simulink model "testPVAsset"  (R2012b)
settings: Solver=FixedStepDiscrete  StartTime=0.0  StopTime=86400  FixedStep=10  RelTol=1e-3
libraries: simulink x1, DiSC_ToolboxOpal_V11 x1
settings Model: Creator=rlo  LastModifiedBy=smartgrid
settings DataIOCC: SignalLoggingSaveFormat=ModelDataLogs
settings OptimizationCC: ExpressionDepthLimit=128
settings DebuggingCC: UnderspecifiedInitializationDetection=Simplified  MergeDetectMultiDrivingBlocksExec=error  MultiTaskDSMMsg=warning  MultiTaskCondExecSysMsg=none  StateNameClashWarn=none  StrictBusMsg=ErrorOnBusTreatedAsVector
settings RTWCC: IncludeERTFirstTime=on
settings CodeAppCC: CustomSymbolStrType=$N$R$M_T  InternalIdentifier=Shortened
settings GRTTargetCC: CodeReplacementLibrary=None  CPPClassGenCompliant=on

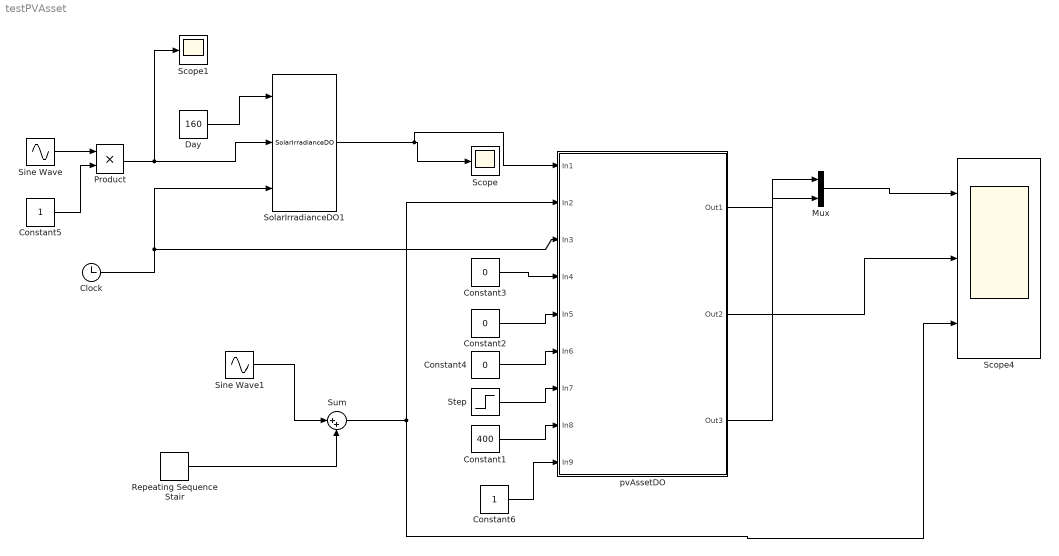
== system testPVAsset ==
  Clock : Clock
  Constant1 : Constant  Value=400
  Constant2 : Constant  Value=0
  Constant3 : Constant  Value=0
  Constant4 : Constant  Value=0
  Constant5 : Constant
  Constant6 : Constant
  Day : Constant  Value=160
  Mux : Mux  Inputs=2
  Product : Product
  Repeating Sequence Stair : simulink/Sources/Repeating Sequence Stair  OutValues="10*[3*ones(1,100)  1*ones(1,100) 4*ones(1,100) 2*ones(1,100) 1*ones(1,100)].'"  tsamp=-1  OutMin=[]  OutMax=[]  OutDataTypeStr=double  OutputDataTypeScalingMode=double  OutDataType=fixdt(0,8)  ConRadixGroup=Best Precision: Vector-wise  OutScaling=2^-12
  Scope : Scope
      settings: YMin=0  YMax=1600
  Scope1 : Scope
      settings: YMin=0  YMax=1
  Scope4 : Scope  NumInputPorts=3
      settings: YMin=0~-5~-5  YMax=6000~5~5  SaveName=ScopeData4
  Sine Wave : Sin  Amplitude=0.5  Bias=0.5  Frequency=0.00004  Phase=pi
  Sine Wave1 : Sin  Amplitude=30  Bias=400  Frequency=0.0001  Phase=pi  SampleTime=0
  SolarIrradianceDO1 : DiSC_ToolboxOpal_V11/SolarIrradianceDO
  Step : Step  Time=0  After=2  SampleTime=0
  Sum : Sum  Inputs=|++
  pvAssetDO : Subsystem
      mask help:
      | %pvAssetDO implements a simple P,Q controllable solar PV system using MATLAB embedded function.
      |     %   The pvAsset can be set to follow an active power reference, output
      |     %   maximum power available or derate power. It can also, at the same
      |     %   time be set to follow a reactive power reference, output the
      |     %   minimum reactive power according to the power factor or try to keep
      |     %   a voltage reference in the coupling point by controlling reactive
      |     %   power output.
      |     %
      |     %
      |     % Revision:
      |     % 19-06-2014, R. Pedersen, Aalborg University. Notes:
      |     % R. Pedersen 11-6-2014, Aalborg University
      |     % 29-11-2014, R. Olsen/M. Kemal, Aalborg University (Simulink)
      |     % 20-06-2015, F. Iov/M. Kemal, Aalborg University (Simulink toolbox for OPAL)
      |
      |                 % Input:
      |             %   - s [w/m^2], is the solar irradiance.
      |             %   - v [V], is the voltage at the connection point.
      |             %   - dP [PU], is the reference to active power change (curtailment).
      |             %   - dPlim [PU], is the reference to derated power (derate)
      |             %   - qRef [VAR], is the reactive power reference.
      |             %   - vRef [V], is the voltage reference.
      |             %
      |             % Output:
      |             %   - p [W], is the active power output
      |             %   - q [VAR], is the reactive power output
      |             %   - pAva [W], is the available power
      mask Help:
      | %pvAssetDO implements a simple P,Q controllable solar PV system using MATLAB embedded function.
      |     %   The pvAsset can be set to follow an active power reference, output
      |     %   maximum power available or derate power. It can also, at the same
      |     %   time be set to follow a reactive power reference, output the
      |     %   minimum reactive power according to the power factor or try to keep
      |     %   a voltage reference in the coupling point by controlling reactive
      |     %   power output.
      |     %
      |     %
      |     % Revision:
      |     % 19-06-2014, R. Pedersen, Aalborg University. Notes:
      |     % R. Pedersen 11-6-2014, Aalborg University
      |     % 29-11-2014, R. Olsen/M. Kemal, Aalborg University (Simulink)
      |     % 20-06-2015, F. Iov/M. Kemal, Aalborg University (Simulink toolbox for OPAL)
      | 
      |                 % Input:
      |             %   - s [w/m^2], is the solar irradiance.
      |             %   - v [V], is the voltage at the connection point.
      |             %   - dP [W], is the reference to active power change.
      |             %   - dPlim [W], is the reference to derated power.
      |             %   - qRef [VAR], is the reactive power reference.
      |             %   - vRef [V], is the voltage reference.
      |             %
      |             % Output:
      |             %   - p [W], is the active power output
      |             %   - q [VAR], is the reactive power output
      |             %   - pAva [W], is the available power
      mask Display:
      | image(imread( 'PhotoVoltaic.png'))
      | port_label( 'output',1, 'p')
      | port_label( 'output',2, 'q')
      | port_label( 'output',3, 'pAva')
      | 
      | 
      | port_label( 'input',1, 'solarIrr')
      | port_label( 'input',2, 'vMeas')
      | port_label( 'input',3, 'time')
      | port_label( 'input',4, 'dp')
      | port_label( 'input',5, 'dplim')
      | port_label( 'input',6, 'qRef')
      | port_label( 'input',7, 'qMode')
      | port_label( 'input',8, 'vRef')
      | port_label( 'input',9, 'pMode')
  wires:
  SolarIrradianceDO1/1 -> pvAssetDO/1(In1), Scope/1
  Day/1 -> SolarIrradianceDO1/1
  Clock/1 -> pvAssetDO/3(In3), SolarIrradianceDO1/3
  Sine Wave/1 -> Product/1
  Product/1 -> SolarIrradianceDO1/2, Scope1/1
  Constant5/1 -> Product/2
  Constant3/1 -> pvAssetDO/4(In4)
  Constant2/1 -> pvAssetDO/5(In5)
  Constant4/1 -> pvAssetDO/6(In6)
  Step/1 -> pvAssetDO/7(In7)
  Constant1/1 -> pvAssetDO/8(In8)
  Constant6/1 -> pvAssetDO/9(In9)
  pvAssetDO/3(Out3) -> Mux/1
  pvAssetDO/1(Out1) -> Mux/2
  Mux/1 -> Scope4/1
  pvAssetDO/2(Out2) -> Scope4/2
  Sine Wave1/1 -> Sum/1
  Sum/1 -> Scope4/3, pvAssetDO/2(In2)
  Repeating Sequence Stair/1 -> Sum/2

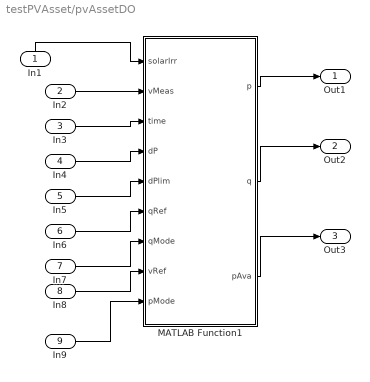
== system testPVAsset/pvAssetDO ==
  In1 : Inport
  In2 : Inport  Port=2
  In3 : Inport  Port=3
  In4 : Inport  Port=4
  In5 : Inport  Port=5
  In6 : Inport  Port=6
  In7 : Inport  Port=7
  In8 : Inport  Port=8
  In9 : Inport  Port=9
  MATLAB Function1 : MATLAB Function  TreatAsAtomicUnit=on
  Out1 : Outport
  Out2 : Outport  Port=2
  Out3 : Outport  Port=3
  wires:
  In6/1 -> MATLAB Function1/6(qRef)
  In5/1 -> MATLAB Function1/5(dPlim)
  MATLAB Function1/1(p) -> Out1/1
  In2/1 -> MATLAB Function1/2(vMeas)
  In4/1 -> MATLAB Function1/4(dP)
  In3/1 -> MATLAB Function1/3(time)
  In1/1 -> MATLAB Function1/1(solarIrr)
  MATLAB Function1/2(q) -> Out2/1
  In8/1 -> MATLAB Function1/8(vRef)
  In7/1 -> MATLAB Function1/7(qMode)
  MATLAB Function1/3(pAva) -> Out3/1
  In9/1 -> MATLAB Function1/9(pMode)

== matlab function testPVAsset/pvAssetDO/MATLAB Function1 ==
  data: solarIrr input; p output; vMeas input; time input; dP input; dPlim input; qRef input; qMode input; vRef input; q output; pAva output; pMode input
function [p,q,pAva] = pvAssetDO(solarIrr,vMeas,time,dP,dPlim,qRef,qMode,vRef,pMode)

%#codegen
%pvAssetDO implements a simple P,Q controllable solar PV system using MATLAB embedded function.
    %   The pvAsset can be set to follow an active power reference, output
    %   maximum power available or derate power. It can also, at the same
    %   time be set to follow a reactive power reference, output the
    %   minimum reactive power according to the power factor or try to keep
    %   a voltage reference in the coupling point by controlling reactive
    %   power output.
    %   
    %   
    % Revision:
    % 19-06-2014, R. Pedersen, Aalborg University. Notes:
    % R. Pedersen 11-6-2014, Aalborg University
    % 29-11-2014, R. Olsen/M. Kemal, Aalborg University (Simulink)
    % 20-06-2015, F. Iov/M. Kemal, Aalborg University (Simulink toolbox for OPAL)
    
                % Input:
            %   - s [w/m^2], is the solar irradiance.
            %   - v [V], is the voltage at the connection point.
            %   - dP [PU], is the reference to active power change (curtailment).
            %   - dPlim [PU], is the reference to derated power (derate)
            %   - qRef [VAR], is the reactive power reference.
            %   - vRef [V], is the voltage reference.
            %
            % Output:
            %   - p [W], is the active power output
            %   - q [VAR], is the reactive power output
            %   - pAva [W], is the available power

            
           
        %properties
        param.vBase = 400;                % Voltage base [V].
        param.pRated = 6e3;               % Rated output power [W].
        param.sMax = 6e3;                 % Maximum apparent power [VA].
        param.A = 25;                     % Area of PV cell [m^2].
        param.eta = 0.25;                  % Efficency of cell [-].
        param.PF = 1;                     % Power factor [-].
        param.Ts = 60;                    % Sampling time (set to 0 if not used)
        param.qFun = 1;
        param.vP = 1.05;
        param.kPP = -300;
        param.kQQ = -300;
        param.vLPFTau = 60*10;
        

     %variable properties     
     persistent var;
     if isempty(var) 
        var.t_c = 0;                    %Time of caching
        var.p_c = 0;                    %Cached values
        var.q_c = 0;
        var.pAva_c = 0;
        var.kPV = 0;               % Gain from s to p [-].
        var.Qmode = 0;                  % Reactive power control mode [-].  
        var.Pmode = 0;                  % Reactive power control mode [-].
        var.vLPFOld = param.vBase;
     end

        
        
% Solar to power conversion factor
     var.kPV = param.eta*param.A;
     
           if (param.Ts>0)
               if (time>(var.t_c+param.Ts))
                   [p,q,pAva,varNew] = samplePV(param,var,solarIrr,vMeas,dP,dPlim,qRef,vRef);
                   var=varNew;
                   var.p_c=p;
                   var.q_c=q;
                   var.pAva_c=pAva;
                   var.t_c=time;
                   var.Qmode = qMode;
                   var.Pmode = pMode;
               end
               p=var.p_c;
               q=var.q_c;
               pAva=var.pAva_c;
            else
               [p,q,pAva,varNew] = samplePV(param,var,solarIrr,vMeas,dP,dPlim,qRef,vRef);
               var=varNew;
               var.Qmode = qMode;
               var.Pmode = pMode;
            end              
  end
